simulink model "fig10_69"  (Simulink 8.4)
settings: Solver=ode23s  SolverMode=SingleTasking  StartTime=0.0  StopTime=100.0  RelTol=1e-3  AbsTol=1e-6
values from neighbouring files (symbols this model uses):
  A = [0    1.0000         0         0 ... (first row only)    [fig10_03.m]    (also in fig10_04.m; fig10_12.m; fig10_13.m; fig10_14.m)
  B = [0 ... (first row only)    [fig10_03.m]    (also in fig10_04.m; fig10_12.m; fig10_13.m; fig10_14.m)
  C = [1     0     0     0]    [fig10_03.m]    (also in fig10_04.m; fig10_12.m; fig10_13.m; fig10_14.m)
  D = [0]    [fig10_03.m]    (also in fig10_04.m; fig10_12.m; fig10_13.m; fig10_14.m)
  L = place(A',C',pe)'    [fig10_21.m]    (also in fig10_22.m; fig10_23.m; fig10_24.m; fig10_37.m = place(Apw',Cpw',pe)')
undefined symbols (not defined in the file or in its folder): K1, Ko
libraries: simulink x1
CloseFcn:
  | ;slview('closediagram',bdroot);
settings Model: Creator=abbas  LastModifiedBy=abbas  ExtModeTrigMode=oneshot  ExtModeArmWhenConnect=off
settings DataIOCC: LimitDataPoints=off
settings OptimizationCC: BlockReduction=off  BooleanDataType=off  InitFltsAndDblsToZero=on
settings DebuggingCC: SaveWithParameterizedLinksMsg=none  SignalResolutionControl=TryResolveAllWithWarning  SolverPrmCheckMsg=none  MultiTaskDSMMsg=warning  MultiTaskCondExecSysMsg=none
settings HardwareCC: TargetUnknown=on
settings RTWCC: IncludeERTFirstTime=on
settings GRTTargetCC: TargetFcnLib=ansi_tfl_tmw.mat  ModelReferenceCompliant=off  CompOptLevelCompliant=off  MatFileLogging=off

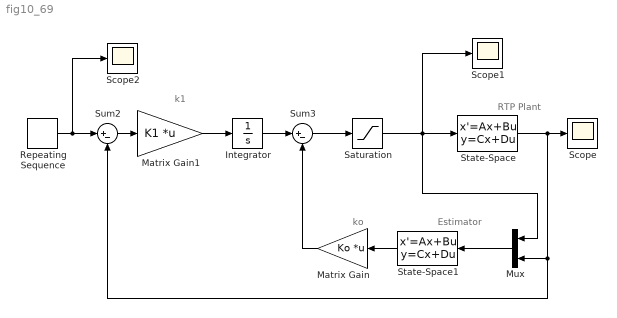
== system fig10_69 ==
  note: ko
  note: k1
  note: Estimator
  note: RTP Plant
  Integrator : Integrator
  Matrix Gain : Gain  Gain=Ko  Multiplication=Matrix(K*u)  SaturateOnIntegerOverflow=on  OutDataTypeStr=Inherit: Same as input  ParamDataTypeStr=Inherit: Same as input
  Matrix Gain1 : Gain  Gain=K1  Multiplication=Matrix(K*u)  SaturateOnIntegerOverflow=on  OutDataTypeStr=Inherit: Same as input  ParamDataTypeStr=Inherit: Same as input
  Mux : Mux  Inputs=2
  Repeating Sequence : simulink/Sources/Repeating Sequence  rep_seq_t=[0:0.1:100]  rep_seq_y=[0:.1:25 25*ones(1,500) 0*ones(1,250)]
  Saturation : Saturate  UpperLimit=20  LowerLimit=-20
  Scope : Scope
      settings: TickLabels=on
  Scope1 : Scope
      settings: TickLabels=on
  Scope2 : Scope
      settings: TickLabels=on
  State-Space : StateSpace  A=A  B=B  C=C  D=D  X0=0
  State-Space1 : StateSpace  A=A-L*C  B=[B L]  C=eye(3)  D=0*ones(3,2)  X0=0
  Sum2 : Sum  Inputs=|+-  SaturateOnIntegerOverflow=on  InputSameDT=on  OutDataTypeStr=Inherit: Same as first input
  Sum3 : Sum  Inputs=|+-  SaturateOnIntegerOverflow=on  InputSameDT=on  OutDataTypeStr=Inherit: Same as first input
  wires:
  Matrix Gain1/1 -> Integrator/1
  Integrator/1 -> Sum3/1
  Sum3/1 -> Saturation/1
  Saturation/1 -> State-Space/1, Scope1/1, Mux/1
  Repeating Sequence/1 -> Scope2/1, Sum2/1
  State-Space/1 -> Scope/1, Mux/2, Sum2/2
  State-Space1/1 -> Matrix Gain/1
  Mux/1 -> State-Space1/1
  Matrix Gain/1 -> Sum3/2
  Sum2/1 -> Matrix Gain1/1
